simulink model "lqr_test_NED"  (R2017a)
settings: Solver=ode4  StartTime=0.0  StopTime=15  FixedStep=Ts  RelTol=1e-3  EnableMultiTasking=on
values from neighbouring files (symbols this model uses):
  A_fil = diag(-1/tau*[1 1 1 1 1 1])    [firefly_parameters_NED.m]
  B = [1 1 1 1 1 1 ... (first row only)    [firefly_parameters_NED.m]
  B_fil = diag(1/tau*[1 1 1 1 1 1])    [firefly_parameters_NED.m]
  C_fil = eye(6)    [firefly_parameters_NED.m]
  D_fil = zeros(6,6)    [firefly_parameters_NED.m]
  Euler_e = [0 0 0]'    [lqr_synthesis_NED.m]
  g0 = gra    [lqr_synthesis_NED.m]
  Ib = [Ixx  0   0 ... (first row only)    [lqr_synthesis_NED.m]
  Ki_lqr = [0 0 -0.22360679775 0 0 0.22360679775 0 0 -27.3861278753 0 0 0 ... (16 elements, 4x4)]    [K_lqr.mat]    (also in lqr_synthesis_NED.m = -K(:,13:end))
  KT = 0.00000854858    (= 8.54858e-06)    [firefly_parameters_NED.m]
  Kx_lqr = [0 0 -0.455716935823 0 0 0.442439914989 0 0 -27.0861476332 0 0 0 ... (48 elements, 4x12)]    [K_lqr.mat]    (also in lqr_synthesis_NED.m = K(:,1:12))
  mass = 1.56779    [firefly_parameters_NED.m]
  Omegab_e = [0 0 0]'    [lqr_synthesis_NED.m]
  Po_e = [0 0 -H_e]'    [lqr_synthesis_NED.m]
  T_max = KT*w_max^2    (= 6.00318901352)    [firefly_parameters_NED.m]
  Te = mass*gra/6    [lqr_synthesis_NED.m]
  Ts = 1/60    (= 0.0166666666667)    [lqr_synthesis_NED.m]
  Vb_e = [0 0 0]'    [lqr_synthesis_NED.m]
  ze = 0    [lqr_synthesis_NED.m]
undefined symbols (not defined in the file or in its folder): magnitude
libraries: simulink x1
settings Model: Creator=dtnguyen  LastModifiedBy=ducnguyen
settings DataIOCC: LimitDataPoints=on  SaveFormat=Array
settings OptimizationCC: DefaultParameterBehavior=Inlined  UseFloatMulNetSlope=on  InlineInvariantSignals=on  EfficientFloat2IntCast=on  LifeSpan=inf
settings DebuggingCC: SFUnexpectedBacktrackingDiag=warning  SFNoUnconditionalDefaultTransitionDiag=warning  SFExecutionAtInitializationDiag=none
settings HardwareCC: ProdBitPerPointer=32  ProdBitPerSizeT=32  ProdBitPerPtrDiffT=32  ProdLargestAtomicFloat=None  ProdIntDivRoundTo=Undefined  ProdEndianess=Unspecified  ProdWordSize=32  ProdHWDeviceType=32-bit Generic
settings ModelReferenceCC: PropagateSignalLabelsOutOfModel=off
settings RTWCC: GenerateReport=on  Toolchain=Catkin  BuildConfiguration=Faster Runs  LaunchReport=on  TargetLang=C++  CheckMdlBeforeBuild=Warning
settings GRTTargetCC: TargetLangStandard=C++03 (ISO)  GeneratePreprocessorConditionals=Disable all  MatFileLogging=off  MultiInstanceERTCode=on  CodeInterfacePackaging=C++ class  SupportNonFinite=off
settings ConfigComp: CovMetricSettings=dw  CovHtmlReporting=on  CovSaveCumulativeToWorkspaceVar=on  CovSaveSingleToWorkspaceVar=on  CovExternalEMLEnable=off

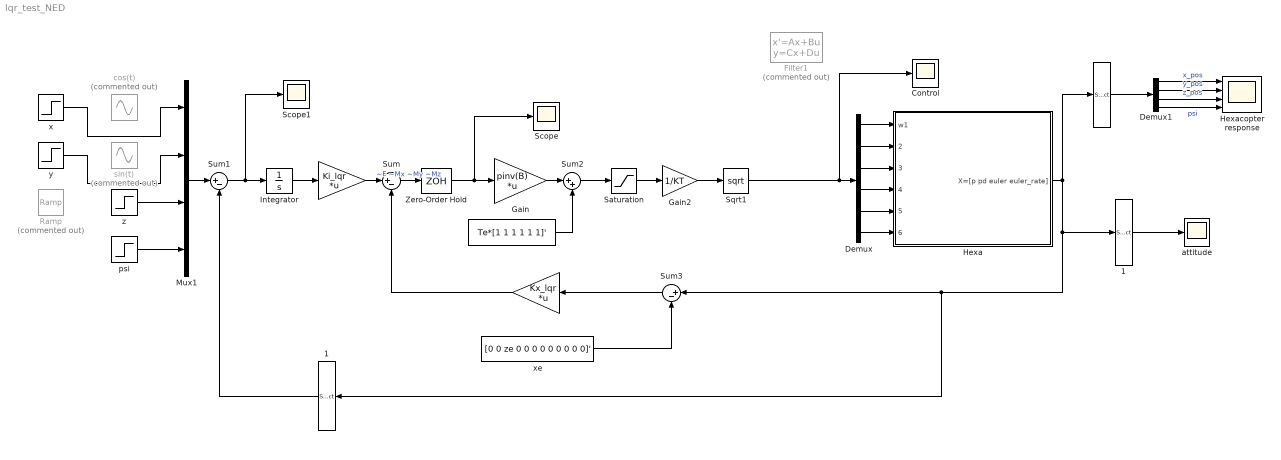
== system lqr_test_NED ==
  " " : Gain  Gain=Ki_lqr  Multiplication=Matrix(K*u)
  "              " : Constant  Value=Te*[1 1 1 1 1 1]'
  "                   " : Gain  Gain=Kx_lqr  Multiplication=Matrix(K*u)
  "                       " : Selector  InputPortWidth=12  IndexOptions=Index vector (dialog)  Indices=[1 2 3 9]  OutputSizes=1
  "                       1" : Selector  InputPortWidth=12  IndexOptions=Index vector (dialog)  Indices=[7 8 9]  OutputSizes=1
  "                    1" : Selector  InputPortWidth=12  IndexOptions=Index vector (dialog)  Indices=[1 2 3 9]  OutputSizes=1
  "              xe" : Constant  Value=[0 0 ze 0 0 0 0 0 0 0 0 0]'
  Control : Scope
  Demux : Demux  Outputs=6
  Demux1 : Demux
  Filter1 : StateSpace  Commented=on  A=A_fil  B=B_fil  C=C_fil  D=D_fil  X0=0
  Gain : Gain  Gain=pinv(B)  Multiplication=Matrix(K*u)
  Gain2 : Gain  Gain=1/KT
  "Hexa " : Subsystem
  Hexacopter response : Scope  NumInputPorts=4
  Integrator : Integrator  InitialCondition=[0 0 -ze*Ts 0]
  Mux1 : Mux
  Ramp : simulink/Sources/Ramp  Commented=on  slope=-0.1  start=5  X0=-2
  Saturation : Saturate  UpperLimit=T_max  LowerLimit=0
  Scope : Scope
  Scope1 : Scope
  Sqrt1 : Sqrt  SaturateOnIntegerOverflow=on
  Sum : Sum  Inputs=|+-
  Sum1 : Sum  Inputs=|+-
  Sum2 : Sum  Inputs=|++
  Sum3 : Sum  Inputs=|+-
  Zero-Order Hold : ZeroOrderHold  SampleTime=-1
  attitude : Scope
  cos(t) : Sin  Commented=on  Amplitude=0  Phase=pi/2  SampleTime=0
  psi : Step  Time=20  After=0  SampleTime=0
  sin(t) : Sin  Commented=on  Amplitude=0  SampleTime=0
  x : Step  Time=5  After=0  SampleTime=0
  y : Step  Time=10  After=0  SampleTime=0
  z : Step  Time=2  After=-1  SampleTime=0
  wires:
  Demux/2 -> "Hexa "/2("  ")
  "Hexa "/1(X=[p pd euler euler_rate]) -> "                       1"/1, Sum3/1, "                    1"/1, "                       "/1
  Demux/5 -> "Hexa "/5("       ")
  Demux/3 -> "Hexa "/3(" ")
  Demux/4 -> "Hexa "/4("    ")
  Demux/6 -> "Hexa "/6("           ")
  Demux/1 -> "Hexa "/1(w1)
  Sum/1 -> Zero-Order Hold/1  "~F ~Mx ~My ~Mz"
  Saturation/1 -> Gain2/1
  "                   "/1 -> Sum/2
  Integrator/1 -> " "/1
  "                    1"/1 -> Sum1/2
  " "/1 -> Sum/1
  Mux1/1 -> Sum1/1
  Gain/1 -> Sum2/1
  "              "/1 -> Sum2/2
  "              xe"/1 -> Sum3/2
  Sum3/1 -> "                   "/1
  Demux1/4 -> Hexacopter response/4  "psi"
  Demux1/2 -> Hexacopter response/2  "y_pos"
  Demux1/1 -> Hexacopter response/1  "x_pos"
  Demux1/3 -> Hexacopter response/3  "z_pos"
  "                       "/1 -> Demux1/1
  z/1 -> Mux1/3
  psi/1 -> Mux1/4
  x/1 -> Mux1/1
  y/1 -> Mux1/2
  "                       1"/1 -> attitude/1
  Sum2/1 -> Saturation/1
  Gain2/1 -> Sqrt1/1
  Sqrt1/1 -> Control/1, Demux/1
  Sum1/1 -> Integrator/1, Scope1/1
  Zero-Order Hold/1 -> Scope/1, Gain/1

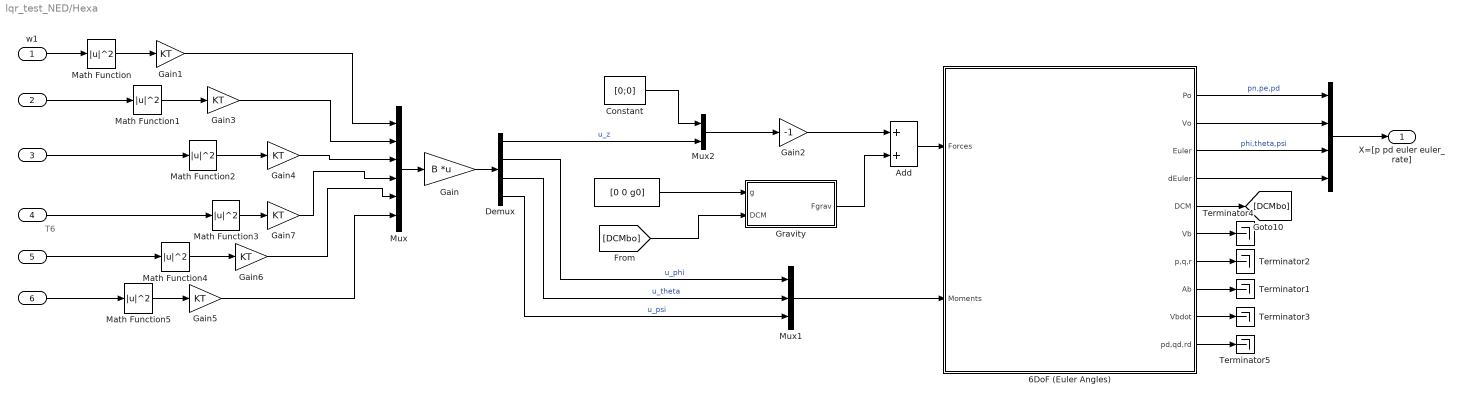
== system lqr_test_NED/Hexa  ==
  note: T6
  w1 : Inport
  "  " : Inport  Port=2
  " " : Inport  Port=3
  "    " : Inport  Port=4
  "       " : Inport  Port=5
  "           " : Inport  Port=6
  "      " : Concatenate  NumInputs=4
  "                  " : Constant  Value=[0 0 g0]
  6DoF (Euler Angles) : Subsystem
  Add : Sum
  Constant : Constant  Value=[0;0]
  Demux : Demux
  Gain : Gain  Gain=B  Multiplication=Matrix(K*u)
  Gain{1,3..7} (6 alike) : Gain  Gain=KT
  Gain2 : Gain  Gain=-1
  "Gravity " : Subsystem
  Math Function{,1..5} (6 alike) : Math  Operator=magnitude^2  SaturateOnIntegerOverflow=on
  Mux : Mux  Inputs=6
  Mux1 : Mux  Inputs=3
  Mux2 : Mux  Inputs=2
  Terminator{1..5} (5 alike) : Terminator
  X=[p pd euler euler_rate] : Outport
  wires:
  Demux/2 -> Mux1/1  "u_phi"
  Demux/3 -> Mux1/2  "u_theta"
  Mux/1 -> Gain/1
  Gain/1 -> Demux/1
  Demux/4 -> Mux1/3  "u_psi"
  Constant/1 -> Mux2/1
  Demux/1 -> Mux2/2  "u_z"
  "                  "/1 -> "Gravity "/1(g)
  "Gravity "/1(Fgrav) -> Add/2
  Add/1 -> 6DoF (Euler Angles)/1(Forces)
  Mux1/1 -> 6DoF (Euler Angles)/2(Moments)
  6DoF (Euler Angles)/9(Vbdot) -> Terminator3/1
  6DoF (Euler Angles)/8(Ab) -> Terminator1/1
  Mux2/1 -> Gain2/1
  Gain2/1 -> Add/1
  "      "/1 -> X=[p pd euler euler_rate]/1
  "       "/1 -> Math Function4/1
  "           "/1 -> Math Function5/1
  "    "/1 -> Math Function3/1
  " "/1 -> Math Function2/1
  "  "/1 -> Math Function1/1
  6DoF (Euler Angles)/1(Po) -> "      "/1  "pn,pe,pd"
  6DoF (Euler Angles)/2(Vo) -> "      "/2
  6DoF (Euler Angles)/3(Euler) -> "      "/3  "phi,theta,psi"
  6DoF (Euler Angles)/4(dEuler) -> "      "/4
  6DoF (Euler Angles)/6(Vb) -> Terminator4/1
  6DoF (Euler Angles)/5(DCM) -> [DCMbo]
  [DCMbo] -> "Gravity "/2(DCM)
  6DoF (Euler Angles)/7(p,q,r) -> Terminator2/1
  6DoF (Euler Angles)/10(pd,qd,rd) -> Terminator5/1
  w1/1 -> Math Function/1
  Math Function/1 -> Gain1/1
  Math Function1/1 -> Gain3/1
  Math Function2/1 -> Gain4/1
  Math Function3/1 -> Gain7/1
  Math Function4/1 -> Gain6/1
  Math Function5/1 -> Gain5/1
  Gain1/1 -> Mux/1
  Gain3/1 -> Mux/2
  Gain4/1 -> Mux/3
  Gain5/1 -> Mux/6
  Gain6/1 -> Mux/5
  Gain7/1 -> Mux/4

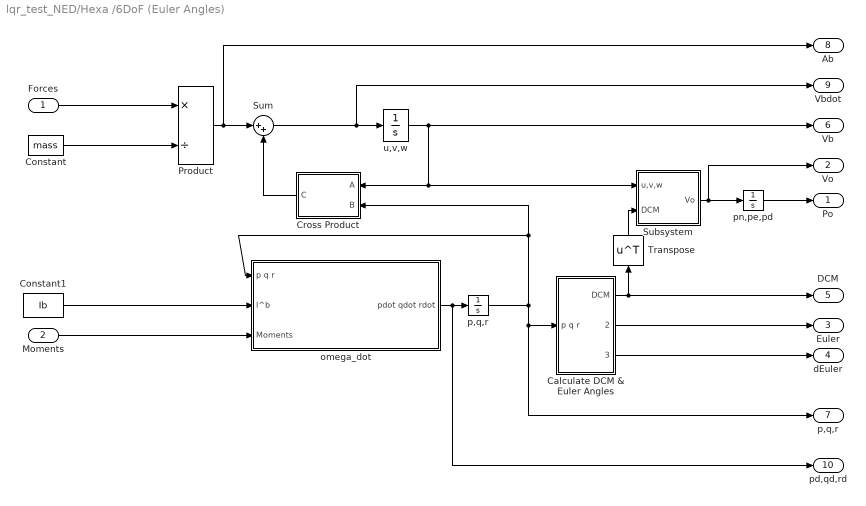
== system lqr_test_NED/Hexa /6DoF (Euler Angles) ==
  Forces : Inport
  Moments : Inport  Port=2
  "Calculate DCM & Euler Angles " : Subsystem
  Constant : Constant  Value=mass  OutDataTypeStr=Inherit: Inherit via back propagation
  Constant1 : Constant  Value=Ib  OutDataTypeStr=Inherit: Inherit via back propagation
  Cross Product : Subsystem
  Product : Product  Inputs=*/  SaturateOnIntegerOverflow=on  OutDataTypeStr=Inherit: Same as first input
  Subsystem : Subsystem
  Sum : Sum  Inputs=|++  SaturateOnIntegerOverflow=on
  Transpose : Math  Operator=transpose  SaturateOnIntegerOverflow=on
  omega_dot : Subsystem
  "p,q,r " : Integrator  InitialCondition=Omegab_e
  pn,pe,pd : Integrator  InitialCondition=Po_e
  u,v,w : Integrator  InitialCondition=Vb_e
  Po : Outport
  Vo : Outport  Port=2
  Euler : Outport  Port=3
  dEuler : Outport  Port=4
  DCM : Outport  Port=5
  Vb : Outport  Port=6
  p,q,r : Outport  Port=7
  Ab : Outport  Port=8
  Vbdot : Outport  Port=9
  pd,qd,rd : Outport  Port=10
  wires:
  Moments/1 -> omega_dot/3(Moments)
  "p,q,r "/1 -> p,q,r/1, "Calculate DCM & Euler Angles "/1("p q r "), Cross Product/2(B), omega_dot/1(p q r)
  Sum/1 -> Vbdot/1, u,v,w/1
  u,v,w/1 -> Vb/1, Cross Product/1(A), Subsystem/1(u,v,w)
  Subsystem/1(Vo) -> Vo/1, pn,pe,pd/1
  pn,pe,pd/1 -> Po/1
  Forces/1 -> Product/1
  Constant/1 -> Product/2
  Transpose/1 -> Subsystem/2(DCM)
  "Calculate DCM & Euler Angles "/1("DCM ") -> Transpose/1, DCM/1
  Product/1 -> Ab/1, Sum/1
  Cross Product/1(C) -> Sum/2
  "Calculate DCM & Euler Angles "/2(Euler) -> Euler/1
  Constant1/1 -> omega_dot/2(I^b)
  omega_dot/1(pdot qdot rdot) -> pd,qd,rd/1, "p,q,r "/1
  "Calculate DCM & Euler Angles "/3(dEuler) -> dEuler/1

== system lqr_test_NED/Hexa /Gravity  ==
  g : Inport
  DCM : Inport  Port=2
  Gravity in Earth Axes : Gain  Gain=mass  SaturateOnIntegerOverflow=on  OutDataTypeStr=Inherit: Same as input  ParamDataTypeStr=Inherit: Same as input
  Inertial to Body : Product  Multiplication=Matrix(*)  SaturateOnIntegerOverflow=on  InputSameDT=on  OutDataTypeStr=Inherit: Same as first input
  Reshape : Reshape  OutputDimensionality=Column vector (2-D)
  Reshape1 : Reshape
  Fgrav : Outport
  wires:
  Inertial to Body/1 -> Reshape1/1
  g/1 -> Gravity in Earth Axes/1
  DCM/1 -> Inertial to Body/1
  Gravity in Earth Axes/1 -> Reshape/1
  Reshape/1 -> Inertial to Body/2
  Reshape1/1 -> Fgrav/1

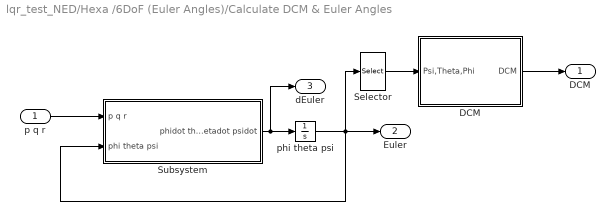
== system lqr_test_NED/Hexa /6DoF (Euler Angles)/Calculate DCM & Euler Angles  ==
  "p q r " : Inport
  DCM : Subsystem
  Selector : Selector  InputPortWidth=3  IndexOptions=Index vector (dialog)  Indices=[3 2 1]  OutputSizes=1
  Subsystem : Subsystem
  phi theta psi : Integrator  InitialCondition=Euler_e
  "DCM " : Outport
  Euler : Outport  Port=2
  dEuler : Outport  Port=3
  wires:
  Selector/1 -> DCM/1(Psi,Theta,Phi)
  phi theta psi/1 -> Subsystem/2(phi theta psi), Euler/1, Selector/1
  Subsystem/1(phidot thetadot psidot) -> dEuler/1, phi theta psi/1
  "p q r "/1 -> Subsystem/1(p q r)
  DCM/1(DCM) -> "DCM "/1

== system lqr_test_NED/Hexa /6DoF (Euler Angles)/Cross Product ==
  A : Inport
  B : Inport  Port=2
  Subsystem : Subsystem
  Subsystem2 : Subsystem
  Sum1 : Sum  Inputs=+|-  SaturateOnIntegerOverflow=on  InputSameDT=on  OutDataTypeStr=Inherit: Same as first input
  C : Outport
  wires:
  A/1 -> Subsystem/1(A), Subsystem2/1(A)
  Subsystem2/1(Out1) -> Sum1/1
  Subsystem/1(Out1) -> Sum1/2
  Sum1/1 -> C/1
  B/1 -> Subsystem/2(B), Subsystem2/2(B)

== system lqr_test_NED/Hexa /6DoF (Euler Angles)/Subsystem ==
  u,v,w : Inport
  DCM : Inport  Port=2
  Product1 : Product  Multiplication=Matrix(*)  SaturateOnIntegerOverflow=on  InputSameDT=on  OutDataTypeStr=Inherit: Same as first input
  Reshape1 : Reshape  OutputDimensionality=Column vector (2-D)
  Reshape2 : Reshape
  Vo : Outport
  wires:
  Reshape2/1 -> Vo/1
  Reshape1/1 -> Product1/2
  u,v,w/1 -> Reshape1/1
  DCM/1 -> Product1/1
  Product1/1 -> Reshape2/1

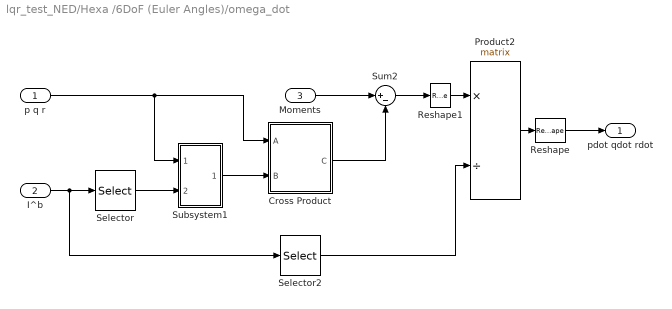
== system lqr_test_NED/Hexa /6DoF (Euler Angles)/omega_dot ==
  p q r : Inport
  I^b : Inport  Port=2
  Moments : Inport  Port=3
  Cross Product : Subsystem
  Product2 : Product  Inputs=*/  Multiplication=Matrix(*)  SaturateOnIntegerOverflow=on  OutDataTypeStr=Inherit: Same as first input
  Reshape : Reshape
  Reshape1 : Reshape  OutputDimensionality=Row vector (2-D)
  Selector : Selector  NumberOfDimensions=2  InputPortWidth=2  IndexOptions=Index vector (dialog),Select all  Indices=1:3,-1  OutputSizes=1
  Selector2 : Selector  NumberOfDimensions=2  InputPortWidth=2  IndexOptions=Index vector (dialog),Select all  Indices=1:3,-1  OutputSizes=1
  Subsystem1 : Subsystem
  Sum2 : Sum  Inputs=|+-  SaturateOnIntegerOverflow=on
  pdot qdot rdot : Outport
  wires:
  I^b/1 -> Selector2/1, Selector/1
  Selector2/1 -> Product2/2
  Selector/1 -> Subsystem1/2(Inertia)
  Reshape/1 -> pdot qdot rdot/1
  Moments/1 -> Sum2/1
  Sum2/1 -> Reshape1/1
  Product2/1 -> Reshape/1
  p q r/1 -> Cross Product/1(A), Subsystem1/1(p q r)
  Reshape1/1 -> Product2/1
  Subsystem1/1(I * w) -> Cross Product/2(B)
  Cross Product/1(C) -> Sum2/2

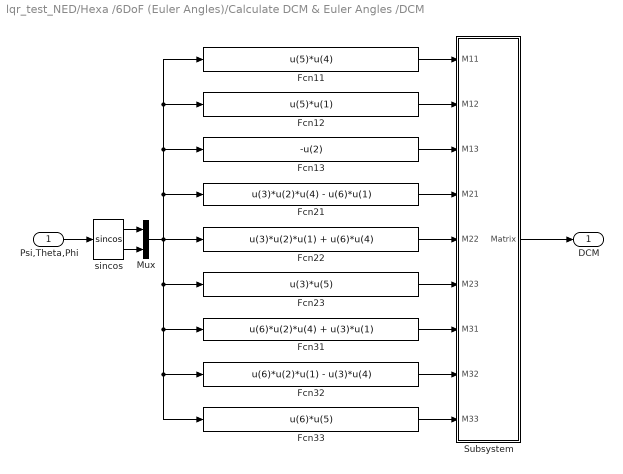
== system lqr_test_NED/Hexa /6DoF (Euler Angles)/Calculate DCM & Euler Angles /DCM ==
  Psi,Theta,Phi : Inport  PortDimensions=3
  Fcn11 : Fcn  Expr=u(5)*u(4)
  Fcn12 : Fcn  Expr=u(5)*u(1)
  Fcn13 : Fcn  Expr=-u(2)
  Fcn21 : Fcn  Expr=u(3)*u(2)*u(4) - u(6)*u(1)
  Fcn22 : Fcn  Expr=u(3)*u(2)*u(1) + u(6)*u(4)
  Fcn23 : Fcn  Expr=u(3)*u(5)
  Fcn31 : Fcn  Expr=u(6)*u(2)*u(4) + u(3)*u(1)
  Fcn32 : Fcn  Expr=u(6)*u(2)*u(1) - u(3)*u(4)
  Fcn33 : Fcn  Expr=u(6)*u(5)
  Mux : Mux  Inputs=2
  Subsystem : Subsystem
  sincos : Trigonometry  Operator=sincos
  DCM : Outport  PortDimensions=[3,3]
  wires:
  Fcn11/1 -> Subsystem/1(M11)
  Fcn12/1 -> Subsystem/2(M12)
  Fcn13/1 -> Subsystem/3(M13)
  Fcn21/1 -> Subsystem/4(M21)
  Fcn31/1 -> Subsystem/7(M31)
  Fcn22/1 -> Subsystem/5(M22)
  Fcn23/1 -> Subsystem/6(M23)
  Fcn32/1 -> Subsystem/8(M32)
  Fcn33/1 -> Subsystem/9(M33)
  Psi,Theta,Phi/1 -> sincos/1
  Subsystem/1(Matrix) -> DCM/1
  sincos/1 -> Mux/1
  sincos/2 -> Mux/2
  Mux/1 -> Fcn11/1, Fcn12/1, Fcn13/1, Fcn21/1, Fcn32/1, Fcn33/1, Fcn31/1, Fcn23/1, Fcn22/1

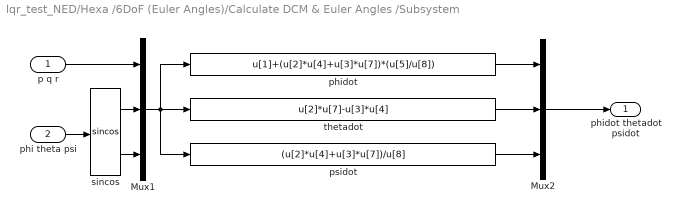
== system lqr_test_NED/Hexa /6DoF (Euler Angles)/Calculate DCM & Euler Angles /Subsystem ==
  p q r : Inport
  phi theta psi : Inport  Port=2
  Mux1 : Mux  Inputs=[3 3 3]
  Mux2 : Mux  Inputs=3
  phidot : Fcn  Expr=u[1]+(u[2]*u[4]+u[3]*u[7])*(u[5]/u[8])
  psidot : Fcn  Expr=(u[2]*u[4]+u[3]*u[7])/u[8]
  sincos : Trigonometry  Operator=sincos
  thetadot : Fcn  Expr=u[2]*u[7]-u[3]*u[4]
  phidot thetadot psidot : Outport
  wires:
  Mux1/1 -> psidot/1, phidot/1, thetadot/1
  p q r/1 -> Mux1/1
  phi theta psi/1 -> sincos/1
  psidot/1 -> Mux2/3
  thetadot/1 -> Mux2/2
  phidot/1 -> Mux2/1
  Mux2/1 -> phidot thetadot psidot/1
  sincos/1 -> Mux1/2
  sincos/2 -> Mux1/3

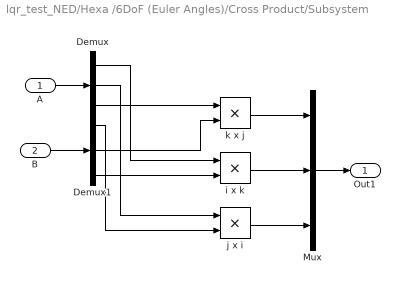
== system lqr_test_NED/Hexa /6DoF (Euler Angles)/Cross Product/Subsystem ==
  A : Inport
  B : Inport  Port=2
  Demux : Demux  Outputs=3
  Demux1 : Demux  Outputs=3
  Mux : Mux  Inputs=3
  i x k : Product  SaturateOnIntegerOverflow=on  InputSameDT=on  OutDataTypeStr=Inherit: Same as first input
  j x i : Product  SaturateOnIntegerOverflow=on  InputSameDT=on  OutDataTypeStr=Inherit: Same as first input
  k x j : Product  SaturateOnIntegerOverflow=on  InputSameDT=on  OutDataTypeStr=Inherit: Same as first input
  Out1 : Outport
  wires:
  j x i/1 -> Mux/3
  i x k/1 -> Mux/2
  k x j/1 -> Mux/1
  Mux/1 -> Out1/1
  Demux1/1 -> j x i/2
  Demux/2 -> j x i/1
  Demux1/3 -> i x k/2
  Demux/1 -> i x k/1
  Demux1/2 -> k x j/2
  Demux/3 -> k x j/1
  B/1 -> Demux1/1
  A/1 -> Demux/1

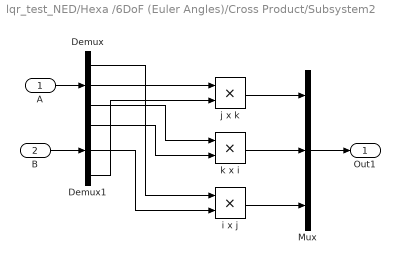
== system lqr_test_NED/Hexa /6DoF (Euler Angles)/Cross Product/Subsystem2 ==
  A : Inport
  B : Inport  Port=2
  Demux : Demux  Outputs=3
  Demux1 : Demux  Outputs=3
  Mux : Mux  Inputs=3
  i x j : Product  SaturateOnIntegerOverflow=on  InputSameDT=on  OutDataTypeStr=Inherit: Same as first input
  j x k : Product  SaturateOnIntegerOverflow=on  InputSameDT=on  OutDataTypeStr=Inherit: Same as first input
  k x i : Product  SaturateOnIntegerOverflow=on  InputSameDT=on  OutDataTypeStr=Inherit: Same as first input
  Out1 : Outport
  wires:
  Demux/3 -> k x i/1
  Demux1/2 -> i x j/2
  k x i/1 -> Mux/2
  i x j/1 -> Mux/3
  Demux/1 -> i x j/1
  Demux1/1 -> k x i/2
  Demux1/3 -> j x k/2
  Mux/1 -> Out1/1
  j x k/1 -> Mux/1
  B/1 -> Demux1/1
  A/1 -> Demux/1
  Demux/2 -> j x k/1

== system lqr_test_NED/Hexa /6DoF (Euler Angles)/omega_dot/Cross Product ==
  A : Inport
  B : Inport  Port=2
  Subsystem : Subsystem
  Subsystem2 : Subsystem
  Sum1 : Sum  Inputs=+|-  SaturateOnIntegerOverflow=on  InputSameDT=on  OutDataTypeStr=Inherit: Same as first input
  C : Outport
  wires:
  A/1 -> Subsystem/1(A), Subsystem2/1(A)
  Subsystem2/1(Out1) -> Sum1/1
  Subsystem/1(Out1) -> Sum1/2
  Sum1/1 -> C/1
  B/1 -> Subsystem/2(B), Subsystem2/2(B)

== system lqr_test_NED/Hexa /6DoF (Euler Angles)/omega_dot/Subsystem1 ==
  p q r : Inport
  Inertia : Inport  Port=2
  Product : Product  Multiplication=Matrix(*)  SaturateOnIntegerOverflow=on  InputSameDT=on  OutDataTypeStr=Inherit: Same as first input
  Reshape2 : Reshape  OutputDimensionality=Column vector (2-D)
  Reshape3 : Reshape
  I * w : Outport
  wires:
  Inertia/1 -> Product/1
  p q r/1 -> Reshape2/1
  Product/1 -> Reshape3/1
  Reshape3/1 -> I * w/1
  Reshape2/1 -> Product/2

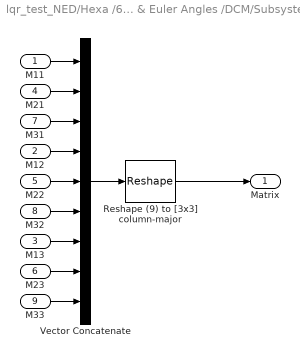
== system lqr_test_NED/Hexa /6DoF (Euler Angles)/Calculate DCM & Euler Angles /DCM/Subsystem ==
  M11 : Inport  PortDimensions=1
  M12 : Inport  Port=2  PortDimensions=1
  M13 : Inport  Port=3  PortDimensions=1
  M21 : Inport  Port=4  PortDimensions=1
  M22 : Inport  Port=5  PortDimensions=1
  M23 : Inport  Port=6  PortDimensions=1
  M31 : Inport  Port=7  PortDimensions=1
  M32 : Inport  Port=8  PortDimensions=1
  M33 : Inport  Port=9  PortDimensions=1
  Reshape (9) to [3x3] column-major : Reshape  OutputDimensionality=Customize  OutputDimensions=[3,3]
  Vector Concatenate : Concatenate  NumInputs=9
  Matrix : Outport  PortDimensions=[3 3]
  wires:
  M32/1 -> Vector Concatenate/6
  Reshape (9) to [3x3] column-major/1 -> Matrix/1
  M22/1 -> Vector Concatenate/5
  M12/1 -> Vector Concatenate/4
  M33/1 -> Vector Concatenate/9
  M23/1 -> Vector Concatenate/8
  M13/1 -> Vector Concatenate/7
  M11/1 -> Vector Concatenate/1
  Vector Concatenate/1 -> Reshape (9) to [3x3] column-major/1
  M31/1 -> Vector Concatenate/3
  M21/1 -> Vector Concatenate/2

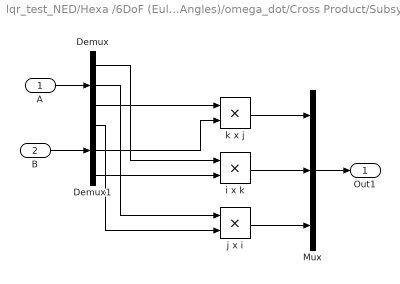
== system lqr_test_NED/Hexa /6DoF (Euler Angles)/omega_dot/Cross Product/Subsystem ==
  A : Inport
  B : Inport  Port=2
  Demux : Demux  Outputs=3
  Demux1 : Demux  Outputs=3
  Mux : Mux  Inputs=3
  i x k : Product  SaturateOnIntegerOverflow=on  InputSameDT=on  OutDataTypeStr=Inherit: Same as first input
  j x i : Product  SaturateOnIntegerOverflow=on  InputSameDT=on  OutDataTypeStr=Inherit: Same as first input
  k x j : Product  SaturateOnIntegerOverflow=on  InputSameDT=on  OutDataTypeStr=Inherit: Same as first input
  Out1 : Outport
  wires:
  j x i/1 -> Mux/3
  i x k/1 -> Mux/2
  k x j/1 -> Mux/1
  Mux/1 -> Out1/1
  Demux1/1 -> j x i/2
  Demux/2 -> j x i/1
  Demux1/3 -> i x k/2
  Demux/1 -> i x k/1
  Demux1/2 -> k x j/2
  Demux/3 -> k x j/1
  B/1 -> Demux1/1
  A/1 -> Demux/1

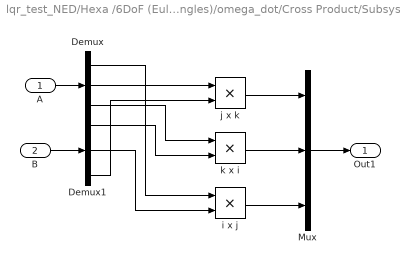
== system lqr_test_NED/Hexa /6DoF (Euler Angles)/omega_dot/Cross Product/Subsystem2 ==
  A : Inport
  B : Inport  Port=2
  Demux : Demux  Outputs=3
  Demux1 : Demux  Outputs=3
  Mux : Mux  Inputs=3
  i x j : Product  SaturateOnIntegerOverflow=on  InputSameDT=on  OutDataTypeStr=Inherit: Same as first input
  j x k : Product  SaturateOnIntegerOverflow=on  InputSameDT=on  OutDataTypeStr=Inherit: Same as first input
  k x i : Product  SaturateOnIntegerOverflow=on  InputSameDT=on  OutDataTypeStr=Inherit: Same as first input
  Out1 : Outport
  wires:
  Demux/3 -> k x i/1
  Demux1/2 -> i x j/2
  k x i/1 -> Mux/2
  i x j/1 -> Mux/3
  Demux/1 -> i x j/1
  Demux1/1 -> k x i/2
  Demux1/3 -> j x k/2
  Mux/1 -> Out1/1
  j x k/1 -> Mux/1
  B/1 -> Demux1/1
  A/1 -> Demux/1
  Demux/2 -> j x k/1
